simulink model "battery_model_closed_loop"  (R2016a)
settings: Solver=VariableStepAuto  StartTime=0.0  StopTime=6000  RelTol=1e-3
values from neighbouring files (symbols this model uses):
  Cnom = 10    [battery_and_controller_parameters.m]
  Crate = 3*Mp*Cnom    (= 90)    [battery_and_controller_parameters.m]
  etaC = 0.995    [battery_and_controller_parameters.m]
  Gc0 = Gcwc*abs(((1/wcp)*(i*wc)^2+(i*wc)))    [battery_and_controller_parameters.m]
  Mp = 3    [battery_and_controller_parameters.m]
  Ns = 100    [battery_and_controller_parameters.m]
  R1 = 5e-3    (= 0.005)    [battery_and_controller_parameters.m]
  Rn = 5e-3    (= 0.005)    [battery_and_controller_parameters.m]
  Rp = 5e-3    (= 0.005)    [battery_and_controller_parameters.m]
  SOC_0 = 0.2    [battery_and_controller_parameters.m]
  SOC_1 = 0.8    [battery_and_controller_parameters.m]
  tau1 = 240    [battery_and_controller_parameters.m]
  tauh = 40    [battery_and_controller_parameters.m]
  Vcell_max = 3.7    [battery_and_controller_parameters.m]
  Vm = 15e-3    (= 0.015)    [battery_and_controller_parameters.m]
  wcp = 2.5*wc    (= 15.7079632679)    [battery_and_controller_parameters.m]
undefined symbols (not defined in the file or in its folder): V_soc
settings Model: Creator=Gorkem  LastModifiedBy=Gorkem

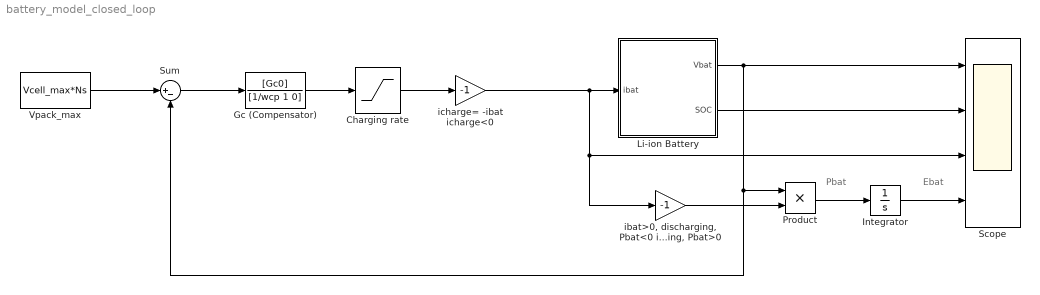
== system battery_model_closed_loop ==
  note: Ebat
  note: Pbat
  Charging rate : Saturate  UpperLimit=Crate  LowerLimit=0
  Gc (Compensator) : TransferFcn  Numerator=[Gc0]  Denominator=[1/wcp 1 0]
  Integrator : Integrator
  Li-ion Battery : Subsystem
  Product : Product
  Scope : Scope  NumInputPorts=4
  Sum : Sum  Inputs=|+-
  Vpack_max : Constant  Value=Vcell_max*Ns
  "ibat>0, discharging, Pbat<0 ibat<0, charging, Pbat>0" : Gain  Gain=-1
  icharge= -ibat icharge<0 : Gain  Gain=-1
  wires:
  Li-ion Battery/2(SOC) -> Scope/2
  icharge= -ibat icharge<0/1 -> "ibat>0, discharging, Pbat<0 ibat<0, charging, Pbat>0"/1, Scope/3, Li-ion Battery/1(ibat)
  Product/1 -> Integrator/1
  "ibat>0, discharging, Pbat<0 ibat<0, charging, Pbat>0"/1 -> Product/2
  Integrator/1 -> Scope/4
  Charging rate/1 -> icharge= -ibat icharge<0/1
  Gc (Compensator)/1 -> Charging rate/1
  Sum/1 -> Gc (Compensator)/1
  Li-ion Battery/1(Vbat) -> Product/1, Sum/2, Scope/1
  Vpack_max/1 -> Sum/1

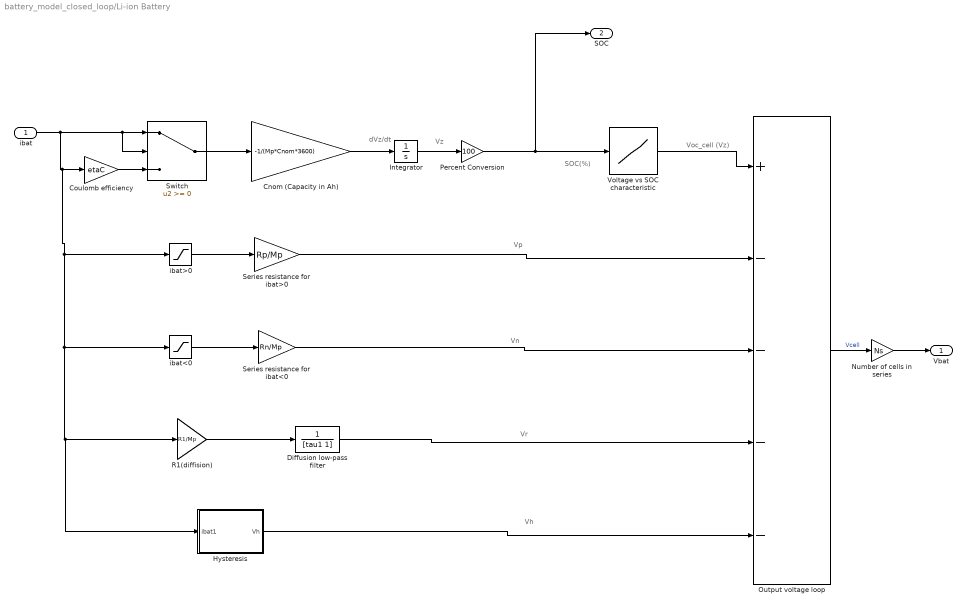
== system battery_model_closed_loop/Li-ion Battery ==
  note: Voc_cell (Vz)
  note: SOC(%)
  note: Vz
  note: Vh
  note: Vr
  note: Vn
  note: Vp
  note: dVz/dt
  ibat : Inport
  Cnom (Capacity in Ah) : Gain  Gain=-1/(Mp*Cnom*3600)
  Coulomb efficiency : Gain  Gain=etaC
  Diffusion low-pass filter : TransferFcn  Denominator=[tau1 1]
  Hysteresis : Subsystem
  Integrator : Integrator  InitialCondition=SOC_0  LimitOutput=on  UpperSaturationLimit=SOC_1  LowerSaturationLimit=0
  Number of cells in series : Gain  Gain=Ns
  Output voltage loop : Sum  Inputs=+----
  "Percent Conversion " : Gain  Gain=100
  R1(diffision) : Gain  Gain=R1/Mp
  Series resistance for ibat<0 : Gain  Gain=Rn/Mp
  Series resistance for ibat>0 : Gain  Gain=Rp/Mp
  Switch : Switch
  Voltage vs SOC characteristic : Lookup_n-D  NumberOfTableDimensions=1  BreakpointsForDimension1=[0:9900]/100  Table=V_soc  InternalRulePriority=Speed  RndMeth=Simplest  InputSameDT=on
  ibat<0 : Saturate  UpperLimit=0  LowerLimit=-inf
  ibat>0 : Saturate  UpperLimit=inf  LowerLimit=0
  Vbat : Outport
  SOC : Outport  Port=2
  wires:
  R1(diffision)/1 -> Diffusion low-pass filter/1
  Diffusion low-pass filter/1 -> Output voltage loop/4
  Series resistance for ibat>0/1 -> Output voltage loop/2
  Integrator/1 -> "Percent Conversion "/1
  "Percent Conversion "/1 -> SOC/1, Voltage vs SOC characteristic/1
  Series resistance for ibat<0/1 -> Output voltage loop/3
  Hysteresis/1(Vh) -> Output voltage loop/5
  ibat/1 -> Hysteresis/1(ibat1), R1(diffision)/1, ibat<0/1, ibat>0/1, Coulomb efficiency/1, Switch/2, Switch/1
  Number of cells in series/1 -> Vbat/1
  Output voltage loop/1 -> Number of cells in series/1  "Vcell"
  Voltage vs SOC characteristic/1 -> Output voltage loop/1
  ibat>0/1 -> Series resistance for ibat>0/1
  Coulomb efficiency/1 -> Switch/3
  Switch/1 -> Cnom (Capacity in Ah)/1
  Cnom (Capacity in Ah)/1 -> Integrator/1
  ibat<0/1 -> Series resistance for ibat<0/1

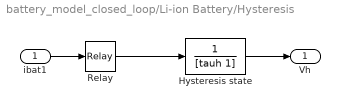
== system battery_model_closed_loop/Li-ion Battery/Hysteresis ==
  ibat1 : Inport
  Hysteresis state : TransferFcn  Denominator=[tauh 1]
  Relay : Relay  OnSwitchValue=0.01  OffSwitchValue=-0.01  OnOutputValue=Vm  OffOutputValue=-Vm
  Vh : Outport
  wires:
  Relay/1 -> Hysteresis state/1
  ibat1/1 -> Relay/1
  Hysteresis state/1 -> Vh/1
